simulink model "autopilota_v_15_last"  (R2020b)
settings: Solver=ode4  StartTime=0.0  StopTime=300  FixedStep=0.02  RelTol=1e-3
values from neighbouring files (symbols this model uses):
  attuatore_Amax = 20*(pi/180)    (= 0.349065850399)    [v2021_10_27_avvioSITL.m]    (also in v2021_10_27_calcoloAerodinamica.m)
  attuatore_Amin = -20*(pi/180)    (= -0.349065850399)    [v2021_10_27_avvioSITL.m]
  attuatore_Emax = 25*(pi/180)    (= 0.436332312999)    [v2021_10_27_avvioSITL.m]    (also in v2021_10_27_calcoloAerodinamica.m)
  attuatore_Emin = -25*(pi/180)    (= -0.436332312999)    [v2021_10_27_avvioSITL.m]
  attuatore_Rmax = 25*(pi/180)    (= 0.436332312999)    [v2021_10_27_avvioSITL.m]    (also in v2021_10_27_calcoloAerodinamica.m)
  attuatore_Rmin = -25*(pi/180)    (= -0.436332312999)    [v2021_10_27_avvioSITL.m]
  attuatore_Tmax = 0.99    [v2021_10_27_avvioSITL.m]
  attuatore_Tmin = 0    [v2021_10_27_avvioSITL.m]
  bias = [baccxINI,baccyINI,bacczINI,bpINI,bqINI,brINI]    [v2021_10_27_avvioSITL.m]
  final_h = 35    [v2021_10_27_avvioSITL.m]
  interventoA_05 = 20*0.8    (= 16)    [v2021_10_27_avvioSITL.m]
  interventoA_1 = 10    [v2021_10_27_avvioSITL.m]
  interventoE_05 = 25*0.8    (= 20)    [v2021_10_27_avvioSITL.m]
  interventoE_1 = 10    [v2021_10_27_avvioSITL.m]
  interventoT = 1*0.6    (= 0.6)    [v2021_10_27_avvioSITL.m]
  inv_A = 1    [v2021_10_27_avvioSITL.m]
  inv_comp_h = 1    [v2021_10_27_avvioSITL.m]
  inv_E = 1    [v2021_10_27_avvioSITL.m]
  inv_R = 1    [v2021_10_27_avvioSITL.m]
  inv_T = 1    [v2021_10_27_avvioSITL.m]
  K_AW_B_AP_quota = 1000    [v2021_10_27_avvioSITL.m]
  K_AW_B_becc = -250    [v2021_10_27_avvioSITL.m]
  K_AW_B_imb = 0    [v2021_10_27_avvioSITL.m]
  K_AW_B_roll = 500    [v2021_10_27_avvioSITL.m]
  K_imb_inv = -0.001306    [v2021_10_27_avvioSITL.m]
  Kd_AP_rotta = 0.995    [v2021_10_27_avvioSITL.m]
  Kd_h_app = 0.085    [v2021_10_27_avvioSITL.m]
  Kd_h_flare = 0.01    [v2021_10_27_avvioSITL.m]
  Ki_AP_quota_select = 0.01936    [v2021_10_27_avvioSITL.m]
  Ki_AP_rotta = 0.002    [v2021_10_27_avvioSITL.m]
  Ki_AP_vel = 0.025175    [v2021_10_27_avvioSITL.m]
  Ki_becch = -0.1963    [v2021_10_27_avvioSITL.m]
  Ki_h_app = 0.055    [v2021_10_27_avvioSITL.m]
  Ki_h_cruise = 0.008    [v2021_10_27_avvioSITL.m]
  Ki_h_flare = 0.07    [v2021_10_27_avvioSITL.m]
  Ki_roll = 0.004528    [v2021_10_27_avvioSITL.m]
  Kp_AP_quota_hold_h = 0.5503    [v2021_10_27_avvioSITL.m]
  Kp_AP_quota_hold_l = 0.5503    [v2021_10_27_avvioSITL.m]
  Kp_AP_quota_select = 0.02647    [v2021_10_27_avvioSITL.m]
  Kp_AP_rotta = 0.520    (= 0.52)    [v2021_10_27_avvioSITL.m]
  Kp_AP_vel = 0.132175    [v2021_10_27_avvioSITL.m]
  Kp_becch = -0.30    (= -0.3)    [v2021_10_27_avvioSITL.m]
  Kp_comp_h = 0.035    [v2021_10_27_avvioSITL.m]
  Kp_h_app_max = 0.086    [v2021_10_27_avvioSITL.m]
  Kp_h_app_min = 0.01    [v2021_10_27_avvioSITL.m]
  Kp_h_cruise = 0.04    [v2021_10_27_avvioSITL.m]
  Kp_h_flare = 0.1    [v2021_10_27_avvioSITL.m]
  Kp_imb = 0.0019415    [v2021_10_27_avvioSITL.m]
  Kp_p = 0.006913    [v2021_10_27_avvioSITL.m]
  Kp_q = -0.025    [v2021_10_27_avvioSITL.m]
  Kp_roll = 0.0718    [v2021_10_27_avvioSITL.m]
  Kp_Rotta_ATO = 4    [v2021_10_27_avvioSITL.m]
  Kp_Rotta_psi = -0.01    [v2021_10_27_avvioSITL.m]
  Q1B = [    2e-15;     2e-15 ... (first row only)    [COV_F1B.m]
  R1B = [     2e-14;             2e-14 ... (first row only)    [COV_F1B.m]
  safe_phi = 55    [v2021_10_27_avvioSITL.m]
  safe_V = 40    [v2021_10_27_avvioSITL.m]
  Sensor_Offsets = [0,0,0]    [v2021_10_27_avvioSITL.m]
  T_cal = 0.4    [v2021_10_27_avvioSITL.m]
  theta_rot = 10    [v2021_10_27_avvioSITL.m]
  time_alarm_SAFE = 300    [v2021_10_27_avvioSITL.m]
  tsamp = 0.02    [v2021_10_27_avvioSITL.m]
  update = [2,2,2]    [v2021_10_27_avvioSITL.m]
  V_max = 35    [v2021_10_27_avvioSITL.m]
  V_stall = 15    [v2021_10_27_avvioSITL.m]
  vd_ini = 0    [v2021_10_27_avvioSITL.m]
  vel_wp1_al = 25    [v2021_10_27_avvioSITL.m]
  vel_wp2_al = 20    [v2021_10_27_avvioSITL.m]
undefined symbols (not defined in the file or in its folder): DiscIntNeverNeededParam, Newton, Raphson, t_AP
libraries: simulink_extras x41, pid_lib x8, dspsigops x4, simulink x3, aerolibtransform2sys x2, aerolibtransform2 x2, cstblocks x1, aerosimlib x1
(part 2 of 11)

== system autopilota_v_15_last/MISURE DA SENSORI FILTRATE/initializer//Clk_generator 1 ==
  Misure : Inport
  calibrating : Inport  Port=2
  Gps_fix_3d : Inport  Port=3
  indice_di_mario : Inport  Port=4
  bias : Inport  Port=5
  Bus Selector2 : BusSelector  Commented=on  OutputSignals=Lat,Long,quota_baro,V_nord,V_est,phi,theta,psi,acc_x,acc_y,acc_z,p,q,r
  Clock GPS1 : Subsystem
  Clock Mti : Subsystem
  Constant : Constant  Value=vd_ini
  Constant1 : Constant
  Constant2 : Constant
  Display : Display
      settings: Decimation=4
  In1 : InportShadow  Port=2
  MATLAB Function2 : MATLAB Function  TreatAsAtomicUnit=on
  Mux2 : Mux  Commented=on  Inputs=14
  Sample and Hold : dspsigops/Sample and Hold  trig=Rising edge  initCond=0  latchinput=off
  Scope2 : Scope  NumInputPorts=3
  Scope3 : Scope  NumInputPorts=2
  Step : Step  Time=T_cal  SampleTime=0.02
  Switch : Switch  Criteria=u2 > Threshold
  Terminator : Terminator
  Cond_ini : Outport  VectorParamsAs1DForOutWhenUnconnected=off
  Enable : Outport  Port=2  VectorParamsAs1DForOutWhenUnconnected=off
  CLock_gps_pos : Outport  Port=3  VectorParamsAs1DForOutWhenUnconnected=off
  "Clock_gps_vel " : Outport  Port=4  VectorParamsAs1DForOutWhenUnconnected=off
  CLock_mti : Outport  Port=5  VectorParamsAs1DForOutWhenUnconnected=off
  wires:
  Gps_fix_3d/1 -> MATLAB Function2/5(fix)
  Clock GPS1/1(clk_pos) -> MATLAB Function2/3(clk_gps), CLock_gps_pos/1, Scope2/2
  Clock Mti/1(Out1) -> Scope2/3, CLock_mti/1, MATLAB Function2/2(clk_ahrs)
  Constant/1 -> MATLAB Function2/6(vd_ini)
  bias/1 -> MATLAB Function2/7(bias)
  indice_di_mario/1 -> Clock GPS1/1(In1)
  Bus Selector2/1 -> Mux2/1  "<Lat>"
  Bus Selector2/2 -> Mux2/2  "<Long>"
  Bus Selector2/3 -> Mux2/3  "<quota_baro>"
  Bus Selector2/4 -> Mux2/4  "<V_nord>"
  Bus Selector2/5 -> Mux2/5  "<V_est>"
  Bus Selector2/6 -> Mux2/6  "<phi>"
  Bus Selector2/7 -> Mux2/7  "<theta>"
  Bus Selector2/8 -> Mux2/8  "<psi>"
  Bus Selector2/9 -> Mux2/9  "<acc_x>"
  Bus Selector2/10 -> Mux2/10  "<acc_y>"
  Bus Selector2/11 -> Mux2/11  "<acc_z>"
  Bus Selector2/12 -> Mux2/12  "<p>"
  Bus Selector2/13 -> Mux2/13  "<q>"
  Bus Selector2/14 -> Mux2/14  "<r>"
  calibrating/1 -> MATLAB Function2/4(Calibrating)
  Step/1 -> Scope3/1
  In1/1 -> Switch/3
  Constant1/1 -> Switch/1
  Switch/1 -> Scope3/2, Enable/1, Sample and Hold/Trigger
  Misure/1 -> Clock Mti/1(In2), Clock GPS1/2(In2), MATLAB Function2/1(misure)
  Clock GPS1/2(clk_vel) -> Scope2/1, "Clock_gps_vel "/1
  MATLAB Function2/1(y) -> Sample and Hold/1
  Sample and Hold/1 -> Display/1, Cond_ini/1
  MATLAB Function2/2(en) -> Terminator/1
  Constant2/1 -> Switch/2

== system autopilota_v_15_last/MISURE DA SENSORI FILTRATE SENZA KALMAN/AOA1 ==
  theta : Inport
  Tas : Inport  Port=2
  RC : Inport  Port=3
  Divide : Product  Inputs=*/
  Sum1 : Sum  Inputs=+-|
  Trigonometric Function : Trigonometry  Operator=asin
  AOA : Outport  VectorParamsAs1DForOutWhenUnconnected=off
  wires:
  theta/1 -> Sum1/1
  Divide/1 -> Trigonometric Function/1
  Sum1/1 -> AOA/1
  Tas/1 -> Divide/2
  Trigonometric Function/1 -> Sum1/2
  RC/1 -> Divide/1

== system autopilota_v_15_last/MISURE DA SENSORI FILTRATE SENZA KALMAN/Subsystem ==
  0-360 : Inport
  Constant : Constant  Value=360
  Sum : Sum  Inputs=|+-
  Switch : Switch  Criteria=u2 > Threshold  Threshold=180
  "+-180 " : Outport  VectorParamsAs1DForOutWhenUnconnected=off
  wires:
  Switch/1 -> "+-180 "/1
  Constant/1 -> Sum/2
  Sum/1 -> Switch/1
  0-360/1 -> Sum/1, Switch/3, Switch/2

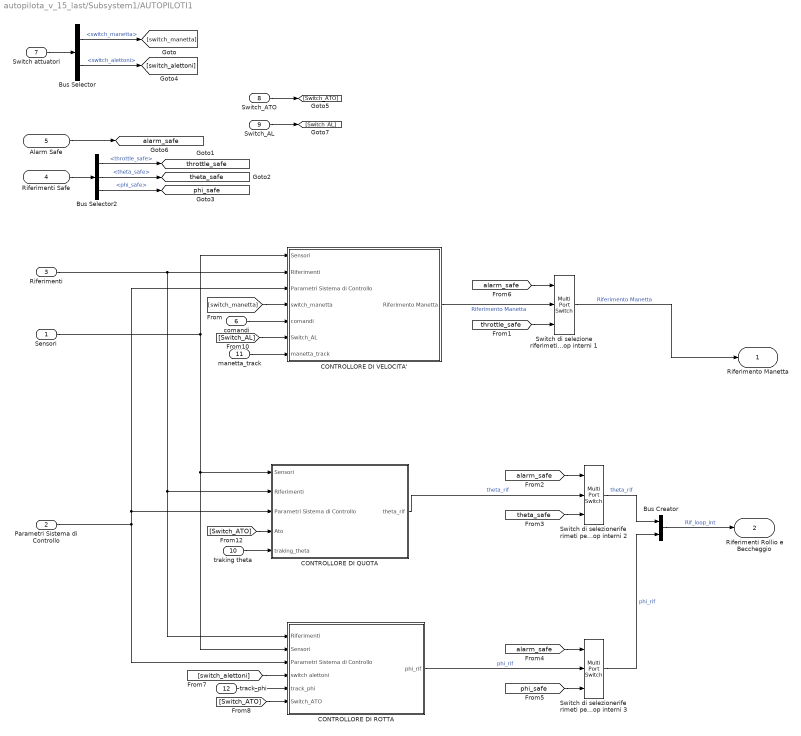
== system autopilota_v_15_last/Subsystem1/AUTOPILOTI1 ==
  Sensori : Inport
  Parametri Sistema di Controllo : Inport  Port=2
  Riferimenti : Inport  Port=3
  Riferimenti Safe : Inport  Port=4
  Alarm Safe : Inport  Port=5
  comandi : Inport  Port=6
  Switch attuatori : Inport  Port=7
  Switch_ATO : Inport  Port=8
  Switch_AL : Inport  Port=9
  traking theta : Inport  Port=10
  manetta_track : Inport  Port=11
  track_phi : Inport  Port=12
  Bus Creator : BusCreator  Inputs=2
  Bus Selector : BusSelector  OutputSignals=switch_manetta,switch_alettoni
  Bus Selector2 : BusSelector  OutputSignals=throttle_safe,theta_safe,phi_safe
  CONTROLLORE DI QUOTA : Subsystem
  CONTROLLORE DI ROTTA : Subsystem
  CONTROLLORE DI VELOCITA' : Subsystem
  Switch di selezione riferimeti per i loop interni 1 : MultiPortSwitch  DataPortOrder=Zero-based contiguous  Inputs=2  zeroidx=on
  Switch di selezioneriferimeti per i loop interni 2 : MultiPortSwitch  DataPortOrder=Zero-based contiguous  Inputs=2  zeroidx=on
  Switch di selezioneriferimeti per i loop interni 3 : MultiPortSwitch  DataPortOrder=Zero-based contiguous  Inputs=2  zeroidx=on
  Riferimento Manetta : Outport  VectorParamsAs1DForOutWhenUnconnected=off
  Riferimenti Rollio e Beccheggio : Outport  Port=2  VectorParamsAs1DForOutWhenUnconnected=off
  tag scope: alarm_safe=global, phi_safe=global, theta_safe=global, throttle_safe=global
  wires:
  Bus Creator/1 -> Riferimenti Rollio e Beccheggio/1  "Rif_loop_int"
  CONTROLLORE DI VELOCITA'/1(Riferimento Manetta) -> Switch di selezione riferimeti per i loop interni 1/2  "Riferimento Manetta"
  Switch di selezione riferimeti per i loop interni 1/1 -> Riferimento Manetta/1  "Riferimento Manetta"
  Switch di selezioneriferimeti per i loop interni 2/1 -> Bus Creator/1  "theta_rif"
  Switch di selezioneriferimeti per i loop interni 3/1 -> Bus Creator/2  "phi_rif"
  [alarm_safe] -> Switch di selezioneriferimeti per i loop interni 2/1
  [alarm_safe] -> Switch di selezioneriferimeti per i loop interni 3/1
  Sensori/1 -> CONTROLLORE DI VELOCITA'/1(Sensori), CONTROLLORE DI ROTTA/2(Sensori), CONTROLLORE DI QUOTA/1(Sensori)
  Riferimenti/1 -> CONTROLLORE DI ROTTA/1(Riferimenti), CONTROLLORE DI QUOTA/2(Riferimenti), CONTROLLORE DI VELOCITA'/2(Riferimenti)
  Parametri Sistema di Controllo/1 -> CONTROLLORE DI VELOCITA'/3(Parametri Sistema di Controllo), CONTROLLORE DI QUOTA/3(Parametri Sistema di Controllo), CONTROLLORE DI ROTTA/3(Parametri Sistema di Controllo)
  Riferimenti Safe/1 -> Bus Selector2/1
  Alarm Safe/1 -> [alarm_safe]
  Bus Selector2/1 -> [throttle_safe]  "<throttle_safe>"
  Bus Selector2/2 -> [theta_safe]  "<theta_safe>"
  Bus Selector2/3 -> [phi_safe]  "<phi_safe>"
  [alarm_safe] -> Switch di selezione riferimeti per i loop interni 1/1
  [throttle_safe] -> Switch di selezione riferimeti per i loop interni 1/3
  [theta_safe] -> Switch di selezioneriferimeti per i loop interni 2/3
  [phi_safe] -> Switch di selezioneriferimeti per i loop interni 3/3
  Switch attuatori/1 -> Bus Selector/1
  Bus Selector/1 -> [switch_manetta]  "<switch_manetta>"
  Bus Selector/2 -> [switch_alettoni]  "<switch_alettoni>"
  comandi/1 -> CONTROLLORE DI VELOCITA'/5(comandi)
  [switch_manetta] -> CONTROLLORE DI VELOCITA'/4(switch_manetta)
  [switch_alettoni] -> CONTROLLORE DI ROTTA/4("switch alettoni ")
  CONTROLLORE DI ROTTA/1(phi_rif) -> Switch di selezioneriferimeti per i loop interni 3/2  "phi_rif"
  Switch_ATO/1 -> [Switch_ATO]
  Switch_AL/1 -> [Switch_AL]
  [Switch_AL] -> CONTROLLORE DI VELOCITA'/6(Switch_AL)
  CONTROLLORE DI QUOTA/1(theta_rif) -> Switch di selezioneriferimeti per i loop interni 2/2  "theta_rif"
  [Switch_ATO] -> CONTROLLORE DI QUOTA/4(Ato)
  traking theta/1 -> CONTROLLORE DI QUOTA/5(traking_theta)
  manetta_track/1 -> CONTROLLORE DI VELOCITA'/7(manetta_track)
  track_phi/1 -> CONTROLLORE DI ROTTA/5(track_phi)
  [Switch_ATO] -> CONTROLLORE DI ROTTA/6(Switch_ATO)

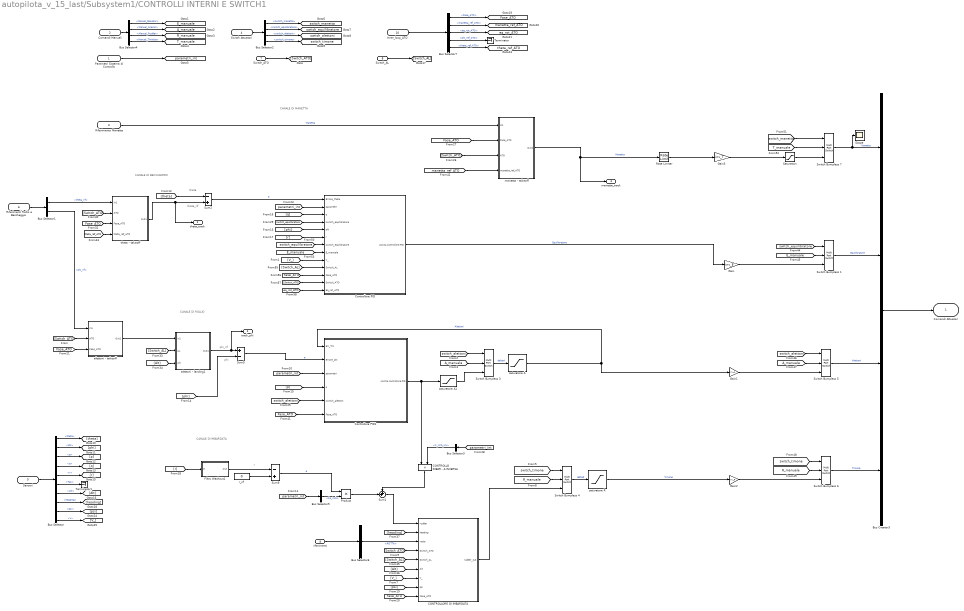
== system autopilota_v_15_last/Subsystem1/CONTROLLI INTERNI E SWITCH1 ==
  note: CANALE DI
      |  MANETTA
  note: theta
  note: theta_rif
  note: CANALE DI
      |  BECCHEGGIO
  note: CANALE
      | DI ROLLIO
  note: CANALE
      | DI IMBARDATA
  note: phi
  note: phi_rif
  note: r
  Parametri Sistema di Controllo : Inport
  Comandi Manuali : Inport  Port=2
  Riferimento Manetta : Inport  Port=3
  Switch Attuatori : Inport  Port=4
  Sensori : Inport  Port=5
  Riferimenti Rollio e Beccheggio : Inport  Port=6
  Switch_ATO : Inport  Port=7
  Switch_AL : Inport  Port=8
  riferimenti : Inport  Port=9
  Inner_loop_ATO : Inport  Port=10
  "  CONTROLLO IMBARDATA INVERSA" : Product  RndMeth=Zero
  Bus Creator3 : BusCreator  Inputs=4
  Bus Selector : BusSelector  OutputSignals=theta,phi,p,q,r,Tas,Alt,heading,psi,v
  Bus Selector1 : BusSelector  OutputSignals=theta_rif,phi_rif
  Bus Selector2 : BusSelector  OutputSignals=switch_manetta,switch_equilibratore,switch_alettoni,switch_timone
  Bus Selector3 : BusSelector  OutputSignals=K_imb_inv
  Bus Selector4 : BusSelector  OutputSignals=Manual_Elevator,Manual_Aileron,Manual_Rudder,Manual_Throttle
  Bus Selector5 : BusSelector  OutputSignals=Kp_imb
  Bus Selector6 : BusSelector  OutputSignals=ROTTA
  Bus Selector7 : BusSelector  OutputSignals=Fase_ATO,manetta_ref_ATO,eq_rot_ATO,phi_ref_ATO,theta_ref_ATO
  CONTROLLORE DI IMBARDATA : Subsystem
  Controllore PID : Subsystem
  Controllore PID1 : Subsystem
  Filtro Washout1 : Subsystem
  Gain : Gain  Gain=inv_E
  Gain1 : Gain  Gain=inv_A
  Gain2 : Gain  Gain=inv_R
  Gain3 : Gain  Gain=inv_T
  Product : Product  RndMeth=Zero
  Rate Limiter : RateLimiter  RisingSlewLimit=0.3  FallingSlewLimit=-0.3  SampleTimeMode=inherited
  Saturation : Saturate  UpperLimit=attuatore_Tmax  LowerLimit=attuatore_Tmin
  Scope : Scope
  Sum1 : Sum  Inputs=++|
  Sum2 : Sum  Inputs=-+
  Sum5 : Sum  Inputs=+-
  Sum9 : Sum  Inputs=-+
  Switch Bumpless {1,3..7} (6 alike) : MultiPortSwitch  DataPortOrder=Zero-based contiguous  Inputs=2  zeroidx=on
  Terminator : Terminator
  Terminator1 : Terminator
  alettoni - landing1 : Subsystem
  alettoni - takeoff : Subsystem
  manetta - takeoff : Subsystem
  r_rif : Constant  Value=0  SampleTime=t_AP
  saturatore A : Saturate  UpperLimit=attuatore_Amax  LowerLimit=attuatore_Amin
  saturatore A1 : Saturate  UpperLimit=attuatore_Amax  LowerLimit=attuatore_Amin
  saturatore R : Saturate  UpperLimit=attuatore_Rmax  LowerLimit=attuatore_Rmin
  theta - takeoff : Subsystem
  Comandi Attuatori : Outport  VectorParamsAs1DForOutWhenUnconnected=off
  theta_track : Outport  Port=2  VectorParamsAs1DForOutWhenUnconnected=off
  manetta_track : Outport  Port=3  VectorParamsAs1DForOutWhenUnconnected=off
  track_phi : Outport  Port=4  VectorParamsAs1DForOutWhenUnconnected=off
  tag scope: A_manuale=global, E_manuale=global, Fase_ATO=global, R_manuale=global, T_manuale=global, eq_rot_ATO=global, manetta_ref_ATO=global, parametri_int=global, switch_alettoni=global, switch_equilibratore=global, switch_manetta=global, switch_timone=global, theta_ref_ATO=global
  wires:
  Comandi Manuali/1 -> Bus Selector4/1
  Bus Selector4/1 -> [E_manuale]  "<Manual_Elevator>"
  Bus Selector4/2 -> [A_manuale]  "<Manual_Aileron>"
  Bus Selector4/3 -> [R_manuale]  "<Manual_Rudder>"
  Bus Selector4/4 -> [T_manuale]  "<Manual_Throttle>"
  Parametri Sistema di Controllo/1 -> [parametri_int]
  Switch Attuatori/1 -> Bus Selector2/1
  Bus Selector2/1 -> [switch_manetta]  "<switch_manetta>"
  Bus Selector2/2 -> [switch_equilibratore]  "<switch_equilibratore>"
  Bus Selector2/3 -> [switch_alettoni]  "<switch_alettoni>"
  Bus Selector2/4 -> [switch_timone]  "<switch_timone>"
  Sensori/1 -> Bus Selector/1
  Riferimenti Rollio e Beccheggio/1 -> Bus Selector1/1
  Bus Selector1/2 -> alettoni - takeoff/1(In1)  "<phi_rif>"
  Switch Bumpless 3/1 -> saturatore A/1  "deltaA"
  saturatore A/1 -> Gain1/1, Controllore PID1/1(Err_Trk)  "Alettoni"
  [switch_alettoni] -> Switch Bumpless 3/1
  [A_manuale] -> Switch Bumpless 3/2
  [switch_timone] -> Switch Bumpless 4/1
  [R_manuale] -> Switch Bumpless 4/2
  r_rif/1 -> Sum9/2
  Filtro Washout1/1(Out) -> Sum9/1
  Bus Creator3/1 -> Comandi Attuatori/1
  Bus Selector3/1 -> "  CONTROLLO IMBARDATA INVERSA"/2  "<K_imb_inv>"
  [parametri_int] -> Bus Selector3/1
  Sum2/1 -> Controllore PID/1(Errore_theta)  "e"
  [switch_equilibratore] -> Controllore PID/4("switch_equilibratore ")
  saturatore A1/1 -> Switch Bumpless 3/3
  [parametri_int] -> Controllore PID/2(parametri)
  [parametri_int] -> Controllore PID1/3(parametri)
  Sum5/1 -> Controllore PID1/2(Errore_phi)  "e"
  Controllore PID1/1(Uscita controllore PID) -> "  CONTROLLO IMBARDATA INVERSA"/1, saturatore A1/1
  saturatore R/1 -> Gain2/1  "Timone"
  Switch Bumpless 4/1 -> saturatore R/1  "deltaR"
  Sum9/1 -> Product/1  "e"
  [parametri_int] -> Bus Selector5/1
  Bus Selector5/1 -> Product/2  "<Kp_imb>"
  Product/1 -> Sum1/2
  Sum1/1 -> CONTROLLORE DI IMBARDATA/1(rudder)
  "  CONTROLLO IMBARDATA INVERSA"/1 -> Sum1/1
  Switch_ATO/1 -> [Switch_ATO]
  Bus Selector/6 -> Terminator1/1  "<Tas>"
  Bus Selector/7 -> [Alt]  "<Alt>"
  alettoni - takeoff/1(Out1) -> alettoni - landing1/1(In1)
  [V_] -> CONTROLLORE DI IMBARDATA/7(V_)
  [Switch_ATO] -> CONTROLLORE DI IMBARDATA/4(Switch_ATO)
  CONTROLLORE DI IMBARDATA/1(rudder_out) -> Switch Bumpless 4/3
  Switch_AL/1 -> [Switch_AL]
  Controllore PID/1(Uscita controllore PID) -> Gain/1  "Equilibratore"
  alettoni - landing1/1(Out1) -> track_phi/1, Sum5/1
  [Switch_AL] -> alettoni - landing1/2(AL)
  [Alt] -> alettoni - landing1/3(Alt)
  [Switch_AL] -> CONTROLLORE DI IMBARDATA/5(Switch_AL)
  [Alt] -> CONTROLLORE DI IMBARDATA/6(Alt)
  riferimenti/1 -> Bus Selector6/1
  Bus Selector6/1 -> CONTROLLORE DI IMBARDATA/3(rotta)  "<ROTTA>"
  [heading] -> CONTROLLORE DI IMBARDATA/2(heading)
  Inner_loop_ATO/1 -> Bus Selector7/1
  Bus Selector7/1 -> [Fase_ATO]  "<Fase_ATO>"
  Bus Selector7/2 -> [manetta_ref_ATO]  "<manetta_ref_ATO>"
  Bus Selector7/3 -> [eq_rot_ATO]  "<eq_rot_ATO>"
  Bus Selector7/4 -> Terminator/1  "<phi_ref_ATO>"
  Bus Selector7/5 -> [theta_ref_ATO]  "<theta_ref_ATO>"
  manetta - takeoff/1(Out1) -> Rate Limiter/1, manetta_track/1  "Manetta"
  Riferimento Manetta/1 -> manetta - takeoff/1(In1)  "Manetta"
  [switch_alettoni] -> Controllore PID1/5("switch_alettoni ")
  [theta] -> Sum2/1
  Bus Selector/1 -> [theta]  "<theta>"
  [phi] -> Controllore PID/5("phi ")
  [phi] -> Sum5/2
  Bus Selector/2 -> [phi]  "<phi>"
  [p] -> Controllore PID1/4("p ")
  Bus Selector/3 -> [p]  "<p>"
  [q] -> Controllore PID/3("q ")
  Bus Selector/4 -> [q]  "<q>"
  [r] -> Controllore PID/6(r)
  [r] -> Filtro Washout1/1(In)
  Bus Selector/5 -> [r]  "<r>"
  Bus Selector/9 -> [psi]  "<psi>"
  [psi] -> CONTROLLORE DI IMBARDATA/8(psi)
  [Fase_ATO] -> CONTROLLORE DI IMBARDATA/9(Fase_ATO)
  [Switch_ATO] -> alettoni - takeoff/2(ATO)
  [Fase_ATO] -> alettoni - takeoff/3(Fase_ATO)
  [Switch_ATO] -> manetta - takeoff/3(ATO)
  [Fase_ATO] -> manetta - takeoff/2(Fase_ATO)
  [manetta_ref_ATO] -> manetta - takeoff/4(manetta_ref_ATO)
  Bus Selector1/1 -> theta - takeoff/1(In1)  "<theta_rif>"
  [Switch_ATO] -> theta - takeoff/2(ATO)
  [Fase_ATO] -> theta - takeoff/3(Fase_ATO)
  [Fase_ATO] -> Controllore PID1/6(Fase_ATO)
  Bus Selector/8 -> [heading]  "<heading>"
  [theta_ref_ATO] -> theta - takeoff/4(theta_ref_ATO)
  Bus Selector/10 -> [V_]  "<v>"
  theta - takeoff/1(Out1) -> theta_track/1, Sum2/2
  Switch Bumpless 1/1 -> Bus Creator3/2  "Equilibratore"
  [E_manuale] -> Switch Bumpless 1/2
  [switch_equilibratore] -> Switch Bumpless 1/1
  Gain/1 -> Switch Bumpless 1/3
  [switch_alettoni] -> Switch Bumpless 5/1
  [A_manuale] -> Switch Bumpless 5/2
  Switch Bumpless 5/1 -> Bus Creator3/3  "Alettoni"
  Gain1/1 -> Switch Bumpless 5/3
  [switch_timone] -> Switch Bumpless 6/1
  [R_manuale] -> Switch Bumpless 6/2
  Switch Bumpless 6/1 -> Bus Creator3/4  "Timone"
  Gain2/1 -> Switch Bumpless 6/3
  [switch_manetta] -> Switch Bumpless 7/1
  [T_manuale] -> Switch Bumpless 7/2
  Switch Bumpless 7/1 -> Scope/1, Bus Creator3/1  "Manetta"
  Gain3/1 -> Saturation/1
  [switch_equilibratore] -> Controllore PID/7(switch_equilibratore)
  [E_manuale] -> Controllore PID/8(E_manuale)
  [Switch_AL] -> Controllore PID/10(Switch_AL)
  [V_] -> Controllore PID/9(V_)
  [Fase_ATO] -> Controllore PID/11(Fase_ATO)
  [Switch_ATO] -> Controllore PID/12(Switch_ATO)
  [eq_rot_ATO] -> Controllore PID/13(Eq_rot_ATO)
  Rate Limiter/1 -> Gain3/1
  Saturation/1 -> Switch Bumpless 7/3

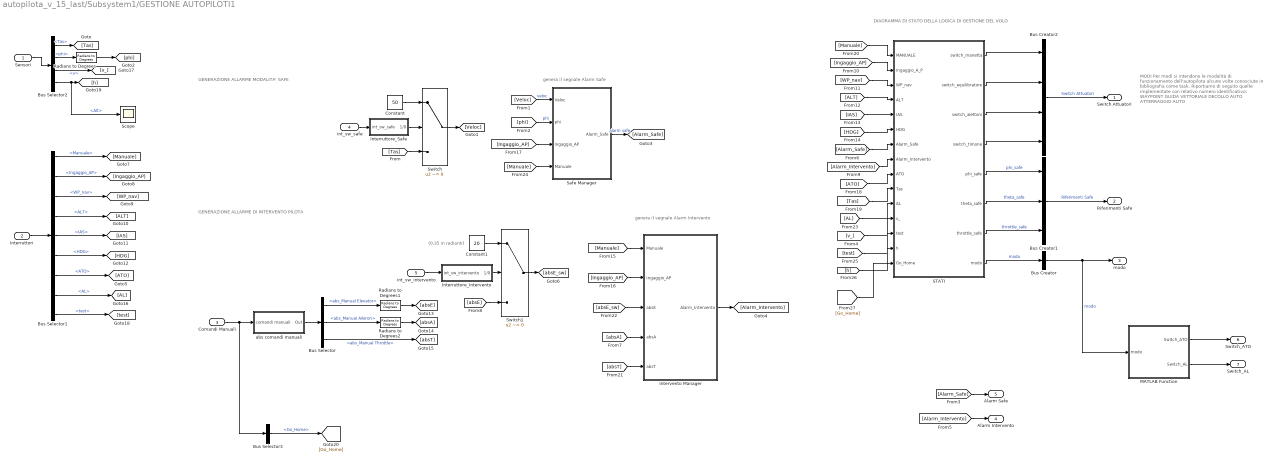
== system autopilota_v_15_last/Subsystem1/GESTIONE AUTOPILOTI1 ==
  note: (0.35 in radianti)
  note: GENERAZIONE ALLARME DI INTERVENTO PILOTA
  note: genera il segnale Alarm Safe
  note: genera il segnale Alarm Intervento
  note: GENERAZIONE ALLARME MODALITA' SAFE
  note: DIAGRAMMA DI STATO
      | DELLA LOGICA DI GESTIONE DEL VOLO
  note: MODI
      | Per modi si intendono le modalità di funzionamento dell'autopilota alcune volte conosciute in bibliografia come task. Riportiamo di seguito quelle implementate con relativo numero identificativo:
      |
      | WAYPOINT
      | GUIDA VETTORIALE
      | DECOLLO AUTO
      | ATTERRAGGIO AUTO
  Sensori : Inport
  "Interruttori " : Inport  Port=2
  Comandi Manuali : Inport  Port=3
  int_sw_safe : Inport  Port=4
  int_sw_intervento : Inport  Port=5
  " STATI" : Stateflow chart  TreatAsAtomicUnit=on
  Bus Creator : BusCreator  Inputs=1
  Bus Creator1 : BusCreator  Inputs=3
  Bus Creator2 : BusCreator  Inputs=4
  Bus Selector : BusSelector  OutputSignals=abs_Manual Elevator,abs_Manual Aileron,abs_Manual Throttle
  Bus Selector1 : BusSelector  OutputSignals=Manuale,Ingaggio_AP,WP_nav,ALT,IAS,HDG,ATO,AL,test
  Bus Selector2 : BusSelector  OutputSignals=Tas,phi,v,Alt
  Bus Selector3 : BusSelector  OutputSignals=Go_Home
  Constant : Constant  Value=50
  Constant1 : Constant  Value=20
  Interruttore_Intervento : Subsystem
  Interruttore_Safe : Subsystem
  Intervento Manager : Subsystem
  MATLAB Function : MATLAB Function  TreatAsAtomicUnit=on
  Radians to Degrees : simulink_extras/Transformations/Radians to Degrees
  Radians to Degrees1 : simulink_extras/Transformations/Radians to Degrees
  Radians to Degrees2 : simulink_extras/Transformations/Radians to Degrees
  Safe Manager : Subsystem
  Scope : Scope
  Switch : Switch  Criteria=u2 ~= 0
  Switch1 : Switch  Criteria=u2 ~= 0
  abs comandi manuali : Subsystem
  Switch Attuatori : Outport  VectorParamsAs1DForOutWhenUnconnected=off
  Riferimenti Safe : Outport  Port=2  VectorParamsAs1DForOutWhenUnconnected=off
  modo : Outport  Port=3  VectorParamsAs1DForOutWhenUnconnected=off
  Alarm Intervento : Outport  Port=4  VectorParamsAs1DForOutWhenUnconnected=off
  Alarm Safe : Outport  Port=5  VectorParamsAs1DForOutWhenUnconnected=off
  Switch_ATO : Outport  Port=6  VectorParamsAs1DForOutWhenUnconnected=off
  Switch_AL : Outport  Port=7  VectorParamsAs1DForOutWhenUnconnected=off
  wires:
  "Interruttori "/1 -> Bus Selector1/1
  Bus Selector1/1 -> [Manuale]  "<Manuale>"
  abs comandi manuali/1(Out) -> Bus Selector/1
  Bus Selector/1 -> Radians to Degrees1/1  "<abs_Manual Elevator>"
  Bus Selector/3 -> [absT]  "<abs_Manual Throttle>"
  Comandi Manuali/1 -> Bus Selector3/1, abs comandi manuali/1(comandi manuali)
  Sensori/1 -> Bus Selector2/1
  Bus Selector1/4 -> [ALT]  "<ALT>"
  Bus Selector1/5 -> [IAS]  "<IAS>"
  Bus Selector1/6 -> [HDG]  "<HDG>"
  Bus Selector2/2 -> Radians to Degrees/1  "<phi>"
  Radians to Degrees/1 -> [phi]
  Bus Selector/2 -> Radians to Degrees2/1  "<abs_Manual Aileron>"
  Bus Selector1/3 -> [WP_nav]  "<WP_nav>"
  Bus Selector2/1 -> [Tas]  "<Tas>"
  Switch/1 -> [Veloc]
  Constant/1 -> Switch/1
  [Tas] -> Switch/3
  [Veloc] -> Safe Manager/1(Veloc)  "veloc"
  Bus Selector1/2 -> [Ingaggio_AP]  "<Ingaggio_AP>"
  [phi] -> Safe Manager/2(phi)  "phi"
  Interruttore_Safe/1(1/0) -> Switch/2
  [Alarm_Safe] -> Alarm Safe/1
  Intervento Manager/1(Alarm_Intervento) -> [Alarm_Intervento]
  [Alarm_Intervento] -> Alarm Intervento/1
  Constant1/1 -> Switch1/1
  [absE] -> Switch1/3
  int_sw_intervento/1 -> Interruttore_Intervento/1(int_sw_intervento)
  Interruttore_Intervento/1(1/0) -> Switch1/2
  [Manuale] -> Intervento Manager/1(Manuale)
  [Ingaggio_AP] -> Intervento Manager/2(Ingaggio_AP)
  [Ingaggio_AP] -> Safe Manager/3(ingaggio_AP)
  [absA] -> Intervento Manager/4(absA)
  int_sw_safe/1 -> Interruttore_Safe/1(int_sw_safe)
  Switch1/1 -> [absE_sw]
  [absE_sw] -> Intervento Manager/3(absE)
  Radians to Degrees1/1 -> [absE]
  Radians to Degrees2/1 -> [absA]
  [absT] -> Intervento Manager/5(absT)
  Bus Selector1/7 -> [ATO]  "<ATO>"
  " STATI"/5(phi_safe) -> Bus Creator1/1  "phi_safe"
  " STATI"/6(theta_safe) -> Bus Creator1/2  "theta_safe"
  " STATI"/7(throttle_safe) -> Bus Creator1/3  "throttle_safe"
  Bus Creator1/1 -> Riferimenti Safe/1  "Riferimenti Safe"
  " STATI"/1(switch_manetta) -> Bus Creator2/1
  " STATI"/2(switch_equilibratore) -> Bus Creator2/2
  " STATI"/3(switch_alettoni) -> Bus Creator2/3
  " STATI"/4(switch_timone) -> Bus Creator2/4
  Bus Creator2/1 -> Switch Attuatori/1  "Switch Attuatori"
  " STATI"/8(modo) -> Bus Creator/1  "modo"
  Bus Creator/1 -> MATLAB Function/1(modo), modo/1  "modo"
  [Alarm_Safe] -> " STATI"/7(Alarm_Safe)
  [Alarm_Intervento] -> " STATI"/8(Alarm_Intervento)
  [Manuale] -> " STATI"/1(MANUALE)
  [Ingaggio_AP] -> " STATI"/2(Ingaggio_A_P)
  [WP_nav] -> " STATI"/3(WP_nav)
  [ALT] -> " STATI"/4(ALT)
  [IAS] -> " STATI"/5(IAS)
  [HDG] -> " STATI"/6(HDG)
  [ATO] -> " STATI"/9(ATO)
  [Tas] -> " STATI"/10(Tas)
  Bus Selector1/8 -> [AL]  "<AL>"
  [AL] -> " STATI"/11(AL)
  Bus Selector2/3 -> [v_]  "<v>"
  [v_] -> " STATI"/12(v_)
  [Manuale] -> Safe Manager/4(Manuale)
  Bus Selector1/9 -> [test]  "<test>"
  [test] -> " STATI"/13(test)
  MATLAB Function/1(Switch_ATO) -> Switch_ATO/1
  MATLAB Function/2(Switch_AL) -> Switch_AL/1
  Bus Selector2/4 -> Scope/1, [h]  "<Alt>"
  [h] -> " STATI"/14(h)
  Bus Selector3/1 -> [Go_Home]  "<Go_Home>"
  [Go_Home] -> " STATI"/15(Go_Home)
  Safe Manager/1(Alarm_Safe) -> [Alarm_Safe]  "alarm safe"

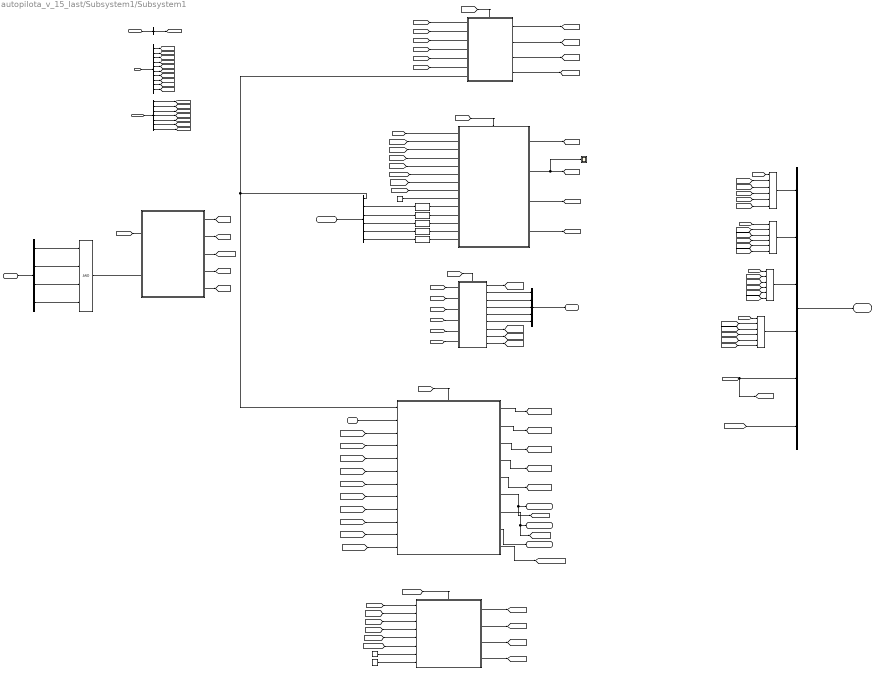
== system autopilota_v_15_last/Subsystem1/Subsystem1 ==
  note: MODO 1 : WAYPOINTS
  note: MODO 2 : VETTORIALE
  note: MODO 3 : DECOLLO AUTO
  note: MODO 4 : ATTERRAGGIO AUTO
  note: MODO 5 : GO HOME
  sensori : Inport
  Interruttori : Inport  Port=2
  waypoints e riferimenti vettoriali : Inport  Port=3
  modo : Inport  Port=4
  Cal_Home : Inport  Port=5
  Switch_attuatori : Inport  Port=6
  AND : Logic  Inputs=4  IconShape=distinctive  AllPortsSameDT=off  OutDataTypeStr=boolean
  Bus Creator : BusCreator  Inputs=5
  Bus Creator2 : BusCreator  Inputs=6
  Bus Selector : BusSelector  OutputSignals=Lat,Long,Alt,psi,heading,Tas,v,theta,RC,quota_lidar
  Bus Selector1 : BusSelector  OutputSignals=GC_info,IAS,ALT,HDG,RC,Ingaggio_AP
  Bus Selector2 : BusSelector  OutputSignals=WP_db_param,WP_db_info,ROTTA,VELOCITA,QUOTA,RC,WP_AL
  Bus Selector3 : BusSelector  OutputSignals=modo
  Bus Selector4 : BusSelector  OutputSignals=switch_manetta,switch_equilibratore,switch_alettoni,switch_timone
  Chart : Stateflow chart  TreatAsAtomicUnit=on
  Constant : Constant  Value=70
  Constant1 : Constant  Value=20
  DECOLLO AUTOMATICO : Subsystem
  Data Type Conversion{,1..4} (5 alike) : DataTypeConversion  OutDataTypeStr=uint8
  RC_default : Constant  Value=2  SampleTime=t_AP
  Scope : Scope
  Subsystem : Subsystem
  Subsystem1 : Subsystem
  Subsystem2 : Subsystem
  Subsystem3 : Subsystem
  Switch di selezione Task - Waypoint navigation{,1..3} (4 alike) : MultiPortSwitch  Inputs=5
  Riferimenti : Outport  VectorParamsAs1DForOutWhenUnconnected=off
  Inner_loop_ATO : Outport  Port=2  VectorParamsAs1DForOutWhenUnconnected=off
  H_LAT : Outport  Port=3  VectorParamsAs1DForOutWhenUnconnected=off
  H_LONG : Outport  Port=4  VectorParamsAs1DForOutWhenUnconnected=off
  H_ALT : Outport  Port=5  VectorParamsAs1DForOutWhenUnconnected=off
  tag scope: modo=global, selector_AL=global
  wires:
  waypoints e riferimenti vettoriali/1 -> Bus Selector2/1
  Bus Selector2/3 -> [ROTTA]  "<ROTTA>"
  Bus Selector2/4 -> [VELOCITA]  "<VELOCITA>"
  Bus Selector2/5 -> [QUOTA]  "<QUOTA>"
  Bus Selector2/6 -> [RC]  "<RC>"
  modo/1 -> Bus Selector3/1
  Bus Selector2/1 -> [WP_db_param]  "<WP_db_param>"
  Bus Selector2/2 -> [WP_db_info]  "<WP_db_info>"
  sensori/1 -> Bus Selector/1
  Bus Selector/1 -> [Lat]  "<Lat>"
  Bus Selector/2 -> [Long]  "<Long>"
  Bus Selector/3 -> [h]  "<Alt>"
  Bus Selector/4 -> [psi]  "<psi>"
  Bus Selector3/1 -> [modo]  "<modo>"
  Bus Selector/6 -> [Tas]  "<Tas>"
  [Tas] -> DECOLLO AUTOMATICO/1(Tas)
  DECOLLO AUTOMATICO/1(rotta_ATO) -> [rotta_ATO]
  DECOLLO AUTOMATICO/7(h_ref_ATO) -> [h_ATO]
  DECOLLO AUTOMATICO/9(RC_ref_ATO) -> [RC_ATO]
  DECOLLO AUTOMATICO/8(Tas_ref_ATO) -> [V_ATO]
  Interruttori/1 -> Bus Selector1/1
  Bus Selector2/7 -> [WP_AL]  "<WP_AL>"
  Bus Selector/7 -> [V_]  "<v>"
  Switch di selezione Task - Waypoint navigation3/1 -> Bus Creator2/4  "ROTTA"
  Bus Creator2/1 -> Riferimenti/1
  Switch di selezione Task - Waypoint navigation/1 -> Bus Creator2/1  "RC"
  Switch di selezione Task - Waypoint navigation1/1 -> Bus Creator2/2  "VELOCITA"
  [modo] -> Switch di selezione Task - Waypoint navigation/1
  [modo] -> Switch di selezione Task - Waypoint navigation1/1
  [modo] -> Switch di selezione Task - Waypoint navigation2/1
  [modo] -> Switch di selezione Task - Waypoint navigation3/1
  [RC_vett] -> Switch di selezione Task - Waypoint navigation/3
  [V_vett] -> Switch di selezione Task - Waypoint navigation1/3
  [rotta_vett] -> Switch di selezione Task - Waypoint navigation3/3
  [RC_wp] -> Switch di selezione Task - Waypoint navigation/2
  [VELOCITA_wp] -> Switch di selezione Task - Waypoint navigation1/2
  [ROTTA_wp] -> Switch di selezione Task - Waypoint navigation3/2
  [V_ATO] -> Switch di selezione Task - Waypoint navigation1/4
  [RC_ATO] -> Switch di selezione Task - Waypoint navigation/4
  [rotta_ATO] -> Switch di selezione Task - Waypoint navigation3/4
  [RC_AL] -> Switch di selezione Task - Waypoint navigation/5
  [V_AL] -> Switch di selezione Task - Waypoint navigation1/5
  [rotta_AL] -> Switch di selezione Task - Waypoint navigation3/5
  [V_goHome] -> Switch di selezione Task - Waypoint navigation1/6
  [rotta_goHome] -> Switch di selezione Task - Waypoint navigation3/6
  [RC_goHome] -> Switch di selezione Task - Waypoint navigation/6
  Bus Selector/5 -> [heading]  "<heading>"
  Switch di selezione Task - Waypoint navigation2/1 -> Bus Creator2/3  "QUOTA"
  [QUOTA_wp] -> Switch di selezione Task - Waypoint navigation2/2
  [h_vett] -> Switch di selezione Task - Waypoint navigation2/3
  [h_ATO] -> Switch di selezione Task - Waypoint navigation2/4
  [h_AL] -> Switch di selezione Task - Waypoint navigation2/5
  [h_goHome] -> Switch di selezione Task - Waypoint navigation2/6
  [h] -> DECOLLO AUTOMATICO/2(h)
  [modo] -> DECOLLO AUTOMATICO/3(modo)
  [psi] -> DECOLLO AUTOMATICO/4(psi_imu)
  DECOLLO AUTOMATICO/2(Fase_ATO) -> Bus Creator/1  "Fase_ATO"
  DECOLLO AUTOMATICO/3(manetta_ref_ATO) -> Bus Creator/2  "manetta_ref_ATO"
  DECOLLO AUTOMATICO/4(eq_rot_ATO) -> Bus Creator/3  "eq_rot_ATO"
  DECOLLO AUTOMATICO/5(phi_ref_ATO) -> Bus Creator/4  "phi_ref_ATO"
  DECOLLO AUTOMATICO/6(theta_ref_ATO) -> Bus Creator/5  "theta_ref_ATO"
  Bus Creator/1 -> Inner_loop_ATO/1
  Bus Selector/8 -> [theta]  "<theta>"
  [theta] -> DECOLLO AUTOMATICO/5(theta)
  [modo] -> Chart/1(modo)
  [modo] -> Subsystem/1(modo)
  [ROTTA] -> Subsystem/2(rotta)
  [VELOCITA] -> Subsystem/3(velocita)
  [QUOTA] -> Subsystem/4(quota)
  [RC] -> Subsystem/5(RC)
  Bus Selector1/2 -> Data Type Conversion/1  "<IAS>"
  [heading] -> Subsystem/6(heading)
  Bus Selector1/3 -> Data Type Conversion1/1  "<ALT>"
  Bus Selector1/4 -> Data Type Conversion2/1  "<HDG>"
  [Tas] -> Subsystem/7(TAS)
  Bus Selector1/5 -> Data Type Conversion3/1  "<RC>"
  [h] -> Subsystem/8(h)
  Bus Selector1/6 -> Data Type Conversion4/1  "<Ingaggio_AP>"
  RC_default/1 -> Subsystem/9(RC_default)
  Subsystem/1(Out1) -> [V_vett]
  Subsystem/2(Out2) -> Scope/1, [h_vett]
  Subsystem/3(Out3) -> [rotta_vett]
  Subsystem/4(Out4) -> [RC_vett]
  Chart/4(Vec_selector) -> [Vec_selector]
  Chart/3(Go_home_selector) -> [Go_home_selector]
  Chart/2(Ato_selector) -> [Ato_selector]
  Chart/1(Al_selector) -> [Al_selector]
  Chart/5(Wp_selector) -> [Wp_selector]
  [Vec_selector] -> Subsystem/Enable
  [Lat] -> Subsystem2/1(In1)
  [Long] -> Subsystem2/2(In2)
  [h] -> Subsystem2/3(In3)
  [psi] -> Subsystem2/4(In4)
  [WP_db_info] -> Subsystem2/5(In5)
  [WP_db_param] -> Subsystem2/6(In6)
  Subsystem2/1(RC) -> [RC_wp]
  Subsystem2/2(VELOCITA) -> [VELOCITA_wp]
  Subsystem2/3(Out3) -> [QUOTA_wp]
  Subsystem2/4(Out4) -> [ROTTA_wp]
  [Wp_selector] -> Subsystem2/Enable
  [Ato_selector] -> DECOLLO AUTOMATICO/Enable
  [Lat] -> Subsystem3/1(In1)
  [Long] -> Subsystem3/2(In2)
  [h] -> Subsystem3/3(In3)
  [psi] -> Subsystem3/4(In4)
  [Lat_Home] -> Subsystem3/5(In5)
  [Long_Home] -> Subsystem3/6(In6)
  Constant/1 -> Subsystem3/7(In7)
  Constant1/1 -> Subsystem3/8(In8)
  Subsystem3/1(Out1) -> [V_goHome]
  Subsystem3/2(Out2) -> [h_goHome]
  Subsystem3/3(Out3) -> [RC_goHome]
  Subsystem3/4(Out4) -> [rotta_goHome]
  [Go_home_selector] -> Subsystem3/Enable
  Switch_attuatori/1 -> Bus Selector4/1
  Bus Selector4/1 -> AND/1  "<switch_manetta>"
  Bus Selector4/2 -> AND/2  "<switch_equilibratore>"
  Bus Selector4/4 -> AND/4  "<switch_timone>"
  Bus Selector4/3 -> AND/3  "<switch_alettoni>"
  AND/1 -> Chart/2(Ap_sel)  "Ap_sel"
  Bus Selector/9 -> [RC_sens]  "<RC>"
  [RC_sens] -> DECOLLO AUTOMATICO/6(RC)
  [Lat] -> Subsystem1/3(Lat)
  Subsystem1/5(landing_selector) -> [landing_selector]
  Subsystem1/6(H_LAT) -> [Lat_Home], H_LAT/1
  [h] -> Subsystem1/5(h)
  Subsystem1/1(TAS_AL) -> [V_AL]
  Subsystem1/3(RC_AL) -> [RC_AL]
  [Al_selector] -> Subsystem1/Enable
  Bus Selector1/1 -> Subsystem1/1(<GC_info>), Subsystem2/7(<GC_info>)  "<GC_info>"
  [Long] -> Subsystem1/4(Long)
  Subsystem1/2(QUOTA_AL) -> [h_AL]
  Subsystem1/8(H_ALT) -> H_ALT/1
  [V_] -> Subsystem1/11(V_)
  [modo] -> Subsystem1/9(modo)
  Subsystem1/4(ROTTA_AL) -> [rotta_AL]
  [Tas] -> Subsystem1/10(TAS)
  Subsystem1/7(H_LONG) -> [Long_Home], H_LONG/1
  Cal_Home/1 -> Subsystem1/2(Cal_home)
  [psi] -> Subsystem1/6(psi)
  [WP_db_info] -> Subsystem1/8(wp_db_info)
  [WP_AL] -> Subsystem1/7(wp_al)
  Bus Selector/10 -> [quota_lidar]  "<quota_lidar>"
  [quota_lidar] -> Subsystem1/12(quota_lidar)
  Data Type Conversion/1 -> Subsystem/10(<IAS>)
  Data Type Conversion1/1 -> Subsystem/11(<ALT>)
  Data Type Conversion2/1 -> Subsystem/12(<HDG>)
  Data Type Conversion3/1 -> Subsystem/13(<RC>)
  Data Type Conversion4/1 -> Subsystem/14(<Ingaggio_AP>)
  [landing_selector] -> [selector_AL], Bus Creator2/5  "landing_selector"
  Subsystem1/9(maneuver_selector) -> [maneuver_selector]
  [maneuver_selector] -> Bus Creator2/6

== system autopilota_v_15_last/scalature comandi /AILERON1 ==
  In1 : Inport
  Constant1 : Constant  Value=1503
  Gain : Gain  Gain=9
  Sum : Sum  Inputs=|++  OutDataTypeStr=double
  Out1 : Outport  VectorParamsAs1DForOutWhenUnconnected=off
  wires:
  Gain/1 -> Sum/1
  Constant1/1 -> Sum/2
  In1/1 -> Gain/1
  Sum/1 -> Out1/1

== system autopilota_v_15_last/scalature comandi /ELEVATOR1 ==
  In1 : Inport
  Constant1 : Constant  Value=3007/2
  Gain : Gain  Gain=447/50
  Sum : Sum  Inputs=|++  OutDataTypeStr=double
  Out1 : Outport  VectorParamsAs1DForOutWhenUnconnected=off
  wires:
  Gain/1 -> Sum/1
  Constant1/1 -> Sum/2
  In1/1 -> Gain/1
  Sum/1 -> Out1/1

== system autopilota_v_15_last/scalature comandi /RUDDER6 ==
  In1 : Inport
  Constant1 : Constant  Value=3007/2
  Gain : Gain  Gain=447/50
  Sum : Sum  Inputs=|++  OutDataTypeStr=double
  Out1 : Outport  VectorParamsAs1DForOutWhenUnconnected=off
  wires:
  Gain/1 -> Sum/1
  Constant1/1 -> Sum/2
  In1/1 -> Gain/1
  Sum/1 -> Out1/1

== system autopilota_v_15_last/scalature comandi /THROTTLE1 ==
  In1 : Inport
  Constant : Constant  Value=1100
  Gain : Gain  Gain=800
  Sum : Sum  Inputs=|++  OutDataTypeStr=double
  Out1 : Outport  VectorParamsAs1DForOutWhenUnconnected=off
  wires:
  In1/1 -> Gain/1
  Gain/1 -> Sum/1
  Constant/1 -> Sum/2
  Sum/1 -> Out1/1

== system autopilota_v_15_last/MISURE DA SENSORI FILTRATE/initializer//Clk_generator 1/Clock GPS1 ==
  In1 : Inport
  In2 : Inport  Port=2
  AND : Logic  Commented=on  IconShape=distinctive  AllPortsSameDT=off  OutDataTypeStr=boolean
  Equal1 : RelationalOperator  Operator===  OutDataTypeStr=boolean  RndMeth=Simplest
  From9 : From  Commented=on  GotoTag=mario
  MATLAB Function : MATLAB Function  TreatAsAtomicUnit=on
  MATLAB Function1 : MATLAB Function  TreatAsAtomicUnit=on
  Memory : Memory
  NOT : Logic  Operator=NOT  IconShape=distinctive  AllPortsSameDT=off  OutDataTypeStr=boolean
  NOT1 : Logic  Commented=on  Operator=NOT  IconShape=distinctive  AllPortsSameDT=off  OutDataTypeStr=boolean
  Pulse Generator3 : DiscretePulseGenerator  Commented=on  PulseType=Time based  Period=0.2  PulseWidth=10
  Scope : Scope
  Terminator : Terminator  Commented=on
  clk_pos : Outport  VectorParamsAs1DForOutWhenUnconnected=off
  clk_vel : Outport  Port=2  VectorParamsAs1DForOutWhenUnconnected=off
  wires:
  Equal1/1 -> NOT/1
  NOT/1 -> Scope/1, MATLAB Function1/1(u), MATLAB Function/1(u)
  In2/1 -> Equal1/1, Memory/1
  Memory/1 -> Equal1/2
  In1/1 -> MATLAB Function1/2(mario), MATLAB Function/2(mario)
  From9/1 -> NOT1/1
  Pulse Generator3/1 -> AND/1
  NOT1/1 -> AND/2
  AND/1 -> Terminator/1
  MATLAB Function1/1(y) -> clk_pos/1
  MATLAB Function/1(y) -> clk_vel/1

== system autopilota_v_15_last/MISURE DA SENSORI FILTRATE/initializer//Clk_generator 1/Clock Mti ==
  In2 : Inport
  Equal : RelationalOperator  Operator===  OutDataTypeStr=boolean  RndMeth=Simplest
  MATLAB Function : MATLAB Function  TreatAsAtomicUnit=on
  Memory : Memory
  NOT : Logic  Operator=NOT  IconShape=distinctive  AllPortsSameDT=off  OutDataTypeStr=boolean
  Out1 : Outport  VectorParamsAs1DForOutWhenUnconnected=off
  wires:
  In2/1 -> Memory/1, Equal/1
  Equal/1 -> NOT/1
  Memory/1 -> Equal/2
  MATLAB Function/1(y) -> Out1/1
  NOT/1 -> MATLAB Function/1(u)

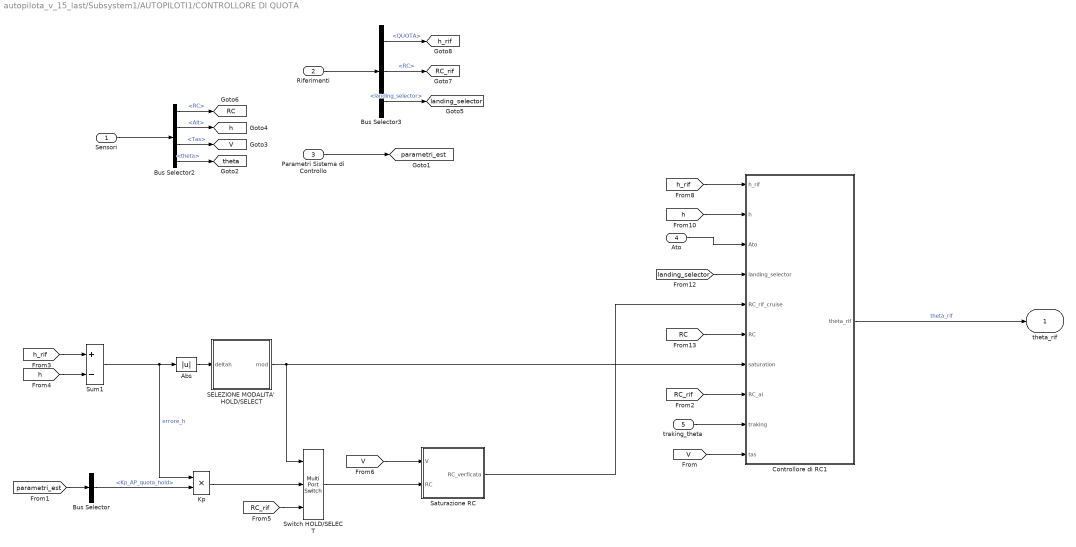
== system autopilota_v_15_last/Subsystem1/AUTOPILOTI1/CONTROLLORE DI QUOTA ==
  Sensori : Inport
  Riferimenti : Inport  Port=2
  Parametri Sistema di Controllo : Inport  Port=3
  Ato : Inport  Port=4
  traking_theta : Inport  Port=5
  Abs : Abs
  Bus Selector : BusSelector  OutputSignals=Kp_AP_quota_hold
  Bus Selector2 : BusSelector  OutputSignals=RC,Alt,Tas,theta
  Bus Selector3 : BusSelector  OutputSignals=QUOTA,RC,landing_selector
  Controllore di RC1 : Subsystem
  Kp : Product  RndMeth=Zero
  SELEZIONE MODALITA' HOLD/SELECT : Stateflow chart  TreatAsAtomicUnit=on
  "Saturazione RC " : Subsystem
  Sum1 : Sum  Inputs=+-
  Switch HOLD/SELECT : MultiPortSwitch  DataPortOrder=Zero-based contiguous  Inputs=2  zeroidx=on
  theta_rif : Outport  VectorParamsAs1DForOutWhenUnconnected=off
  tag scope: RC=global, RC_rif=global, V=global, h=global, h_rif=global, landing_selector=global, parametri_est=global, theta=global
  wires:
  Sensori/1 -> Bus Selector2/1
  Riferimenti/1 -> Bus Selector3/1
  Parametri Sistema di Controllo/1 -> [parametri_est]
  Bus Selector2/1 -> [RC]  "<RC>"
  Bus Selector2/2 -> [h]  "<Alt>"
  Bus Selector2/3 -> [V]  "<Tas>"
  Bus Selector2/4 -> [theta]  "<theta>"
  Bus Selector3/1 -> [h_rif]  "<QUOTA>"
  Bus Selector3/2 -> [RC_rif]  "<RC>"
  [V] -> "Saturazione RC "/1(V)
  Sum1/1 -> Abs/1, Kp/1  "errore_h"
  [h_rif] -> Sum1/1
  [h] -> Sum1/2
  Abs/1 -> SELEZIONE MODALITA' HOLD/SELECT/1(deltah)
  Kp/1 -> Switch HOLD/SELECT/2
  [RC_rif] -> Switch HOLD/SELECT/3
  SELEZIONE MODALITA' HOLD/SELECT/1(mod) -> Switch HOLD/SELECT/1, Controllore di RC1/7(saturation)
  [parametri_est] -> Bus Selector/1
  Bus Selector/1 -> Kp/2  "<Kp_AP_quota_hold>"
  Switch HOLD/SELECT/1 -> "Saturazione RC "/2(RC)
  Bus Selector3/3 -> [landing_selector]  "<landing_selector>"
  [h] -> Controllore di RC1/2(h)
  [h_rif] -> Controllore di RC1/1(h_rif)
  [landing_selector] -> Controllore di RC1/4(landing_selector)
  Ato/1 -> Controllore di RC1/3("Ato ")
  Controllore di RC1/1(theta_rif) -> theta_rif/1  "theta_rif"
  [RC] -> Controllore di RC1/6(RC)
  "Saturazione RC "/1(RC_verficata) -> Controllore di RC1/5(RC_rif_cruise)
  [RC_rif] -> Controllore di RC1/8("RC_al ")
  traking_theta/1 -> Controllore di RC1/9(traking)
  [V] -> Controllore di RC1/10(tas)

== system autopilota_v_15_last/Subsystem1/AUTOPILOTI1/CONTROLLORE DI ROTTA ==
  Riferimenti : Inport
  Sensori : Inport  Port=2
  Parametri Sistema di Controllo : Inport  Port=3
  "switch alettoni " : Inport  Port=4
  track_phi : Inport  Port=5
  Switch_ATO : Inport  Port=6
  ATO : Subsystem
  Bus Selector1 : BusSelector  OutputSignals=ROTTA
  Bus Selector3 : BusSelector  OutputSignals=Kp_AP_rotta,Ki_AP_rotta
  Bus Selector4 : BusSelector  OutputSignals=heading,Tas,phi,Alt,psi,v
  Constant : Constant  Value=70
  Constant2 : Constant  Value=Ki_AP_rotta
  PID Controller1 : pid_lib/PID Controller  Controller=PID  Form=Parallel  TimeDomain=Discrete-time  UseExternalTs=off  SampleTime=-1  IntegratorMethod=Forward Euler  FilterMethod=Forward Euler  ControllerParametersSource=external  P=1  I=1  D=0  UseFilter=on  N=100  TunerSelectOption=Transfer Function Based (PID Tuner App)  InitialConditionSource=internal  InitialConditionForIntegrator=0  InitialConditionForFilter=0  DifferentiatorICPrevScaledInput=0  ExternalReset=none  TrackingMode=on  Kt=1  LimitOutput=on  SatLimitsSource=internal  UpperSaturationLimit=0.7854  LowerSaturationLimit=-0.7854  LinearizeAsGain=on  AntiWindupMode=clamping  Kb=0.1  POutMin=[]  POutMax=[]  IOutMin=[]  IOutMax=[]  DOutMin=[]  DOutMax=[]  NOutMin=[]  NOutMax=[]  SumOutMin=[]  SumOutMax=[]  SaturationOutMin=[]  SaturationOutMax=[]  PParamMin=[]  PParamMax=[]  IParamMin=[]  IParamMax=[]  DParamMin=[]  DParamMax=[]  NParamMin=[]  NParamMax=[]  KbParamMin=[]  KbParamMax=[]  KtParamMin=[]  KtParamMax=[]  KbOutMin=[]  KbOutMax=[]  KtOutMin=[]  KtOutMax=[]  IntegratorOutMin=[]  IntegratorOutMax=[]  FilterOutMin=[]  FilterOutMax=[]  SumI1OutMin=[]  SumI1OutMax=[]  SumI2OutMin=[]  SumI2OutMax=[]  SumI3OutMin=[]  SumI3OutMax=[]  SumI4OutMin=[]  SumI4OutMax=[]  SumDOutMin=[]  SumDOutMax=[]  DifferentiatorOutMin=[]  DifferentiatorOutMax=[]  FilterDiffOutCoefMin=[]  FilterDiffOutCoefMax=[]  ReciprocalOutMin=[]  ReciprocalOutMax=[]  SumDenOutMin=[]  SumDenOutMax=[]  SumNumOutMin=[]  SumNumOutMax=[]  DivideOutMin=[]  DivideOutMax=[]  UdiffTsProdOutMin=[]  UdiffTsProdOutMax=[]  NTsProdOutMin=[]  NTsProdOutMax=[]  UintegralTsProdOutMin=[]  UintegralTsProdOutMax=[]  UngainTsProdOutMin=[]  UngainTsProdOutMax=[]  IntegratorContinuousStateAttributes=''  IntegratorStateMustResolveToSignalObject=off  IntegratorRTWStateStorageClass=Auto  FilterContinuousStateAttributes=''  FilterStateMustResolveToSignalObject=off  FilterRTWStateStorageClass=Auto  ParallelPVariant=ExternalParameters  IdealPVariant=Disabled  IVariant=ExternalParameters  DVariant=ExternalParameters  IntegratorVariant=Discrete  SatVariant=Enabled  AWVariant=DiscClampingParallel  PCopyVariant=Disabled  TRVariant=Enabled  FdbkBlocksVariant=Forward  IdealPFdbkVariant=Disabled  SatFdbkVariant=Disabled  DerivativeFilterVariant=ForwardEulerFilter  NVariant=ExternalParameters  NCopyVariant=Disabled  FilterICVariant=InternalICsFilter  IntegratorICVariant=InternalICs  ExternalResetVariant=Disabled  TRSumVariant=TrackingMode  SumFdbkVariant=Disabled  SumVariant=Sum_PID  TsampFilterVariant=InternalTs  TsampNgainVariant=Passthrough  TsampIntegralVariant=Passthrough  ExternalSaturationOutDataTypeStr=Inherit: Same as second input
  Switch : Switch  Criteria=u2 > Threshold  Threshold=5
  Switch auto-manual : MultiPortSwitch  DataPortOrder=Zero-based contiguous  Inputs=2  zeroidx=on
  Terminator : Terminator
  "calcolo errore Psi " : Subsystem
  phi_rif : Outport  VectorParamsAs1DForOutWhenUnconnected=off
  wires:
  Bus Selector1/1 -> "calcolo errore Psi "/1(psi_ref (°))  "<ROTTA>"
  Sensori/1 -> Bus Selector4/1
  Riferimenti/1 -> Bus Selector1/1
  Bus Selector4/1 -> [heading]  "<heading>"
  Bus Selector4/2 -> Terminator/1  "<Tas>"
  [rotta] -> "calcolo errore Psi "/2(psi (rad))
  Bus Selector4/3 -> [phi]  "<phi>"
  Parametri Sistema di Controllo/1 -> Bus Selector3/1
  "calcolo errore Psi "/1(psi_err) -> PID Controller1/1
  Constant/1 -> PID Controller1/5
  PID Controller1/1 -> Switch auto-manual/3
  Bus Selector4/4 -> [Alt]  "<Alt>"
  Bus Selector3/2 -> ATO/4(In4)  "<Ki_AP_rotta>"
  Bus Selector3/1 -> ATO/1(In1)  "<Kp_AP_rotta>"
  Constant2/1 -> PID Controller1/3
  "switch alettoni "/1 -> Switch auto-manual/1
  Bus Selector4/5 -> [psi]  "<psi>"
  Bus Selector4/6 -> [V_]  "<v>"
  [V_] -> Switch/2
  [heading] -> Switch/1
  [psi] -> Switch/3
  Switch/1 -> [rotta]
  [phi] -> Switch auto-manual/2
  Switch auto-manual/1 -> phi_rif/1
  track_phi/1 -> PID Controller1/6
  [Switch_ATO] -> ATO/2(In2)
  [Alt] -> ATO/3(In3)
  ATO/1(Out1) -> PID Controller1/2
  ATO/2("Out2 ") -> PID Controller1/4
  Switch_ATO/1 -> [Switch_ATO]

== system autopilota_v_15_last/Subsystem1/AUTOPILOTI1/CONTROLLORE DI VELOCITA' ==
  note: CANALE DI
      |  VELOCITA'
  Sensori : Inport
  Riferimenti : Inport  Port=2
  Parametri Sistema di Controllo : Inport  Port=3
  switch_manetta : Inport  Port=4
  comandi : Inport  Port=5
  Switch_AL : Inport  Port=6
  manetta_track : Inport  Port=7
  Bus Selector : BusSelector  OutputSignals=VELOCITA,QUOTA,maneuver selector
  Bus Selector1 : BusSelector  OutputSignals=Tas,Alt,quota_lidar
  Bus Selector2 : BusSelector  OutputSignals=Kp_AP_vel,Ki_AP_vel
  Bus Selector3 : BusSelector  OutputSignals=Manual_Throttle
  PID Controller : pid_lib/PID Controller  Controller=PI  Form=Parallel  TimeDomain=Discrete-time  UseExternalTs=off  SampleTime=-1  IntegratorMethod=Forward Euler  FilterMethod=Forward Euler  ControllerParametersSource=external  P=1  I=1  D=0  UseFilter=on  N=100  TunerSelectOption=Transfer Function Based (PID Tuner App)  InitialConditionSource=internal  InitialConditionForIntegrator=0  InitialConditionForFilter=0  DifferentiatorICPrevScaledInput=0  ExternalReset=none  TrackingMode=on  Kt=1  LimitOutput=on  SatLimitsSource=internal  UpperSaturationLimit=attuatore_Tmax  LowerSaturationLimit=attuatore_Tmin  LinearizeAsGain=on  AntiWindupMode=clamping  Kb=1  POutMin=[]  POutMax=[]  IOutMin=[]  IOutMax=[]  DOutMin=[]  DOutMax=[]  NOutMin=[]  NOutMax=[]  SumOutMin=[]  SumOutMax=[]  SaturationOutMin=[]  SaturationOutMax=[]  PParamMin=[]  PParamMax=[]  IParamMin=[]  IParamMax=[]  DParamMin=[]  DParamMax=[]  NParamMin=[]  NParamMax=[]  KbParamMin=[]  KbParamMax=[]  KtParamMin=[]  KtParamMax=[]  KbOutMin=[]  KbOutMax=[]  KtOutMin=[]  KtOutMax=[]  IntegratorOutMin=[]  IntegratorOutMax=[]  FilterOutMin=[]  FilterOutMax=[]  SumI1OutMin=[]  SumI1OutMax=[]  SumI2OutMin=[]  SumI2OutMax=[]  SumI3OutMin=[]  SumI3OutMax=[]  SumI4OutMin=[]  SumI4OutMax=[]  SumDOutMin=[]  SumDOutMax=[]  DifferentiatorOutMin=[]  DifferentiatorOutMax=[]  FilterDiffOutCoefMin=[]  FilterDiffOutCoefMax=[]  ReciprocalOutMin=[]  ReciprocalOutMax=[]  SumDenOutMin=[]  SumDenOutMax=[]  SumNumOutMin=[]  SumNumOutMax=[]  DivideOutMin=[]  DivideOutMax=[]  UdiffTsProdOutMin=[]  UdiffTsProdOutMax=[]  NTsProdOutMin=[]  NTsProdOutMax=[]  UintegralTsProdOutMin=[]  UintegralTsProdOutMax=[]  UngainTsProdOutMin=[]  UngainTsProdOutMax=[]  IntegratorContinuousStateAttributes=''  IntegratorStateMustResolveToSignalObject=off  IntegratorRTWStateStorageClass=Auto  FilterContinuousStateAttributes=''  FilterStateMustResolveToSignalObject=off  FilterRTWStateStorageClass=Auto  ParallelPVariant=ExternalParameters  IdealPVariant=Disabled  IVariant=ExternalParameters  DVariant=Disabled  IntegratorVariant=Discrete  SatVariant=Enabled  AWVariant=DiscClampingParallel  PCopyVariant=Disabled  TRVariant=Enabled  FdbkBlocksVariant=Forward  IdealPFdbkVariant=Disabled  SatFdbkVariant=Disabled  DerivativeFilterVariant=Disabled  NVariant=Disabled  NCopyVariant=Disabled_SignalSpec  FilterICVariant=Disabled  IntegratorICVariant=InternalICs  ExternalResetVariant=Disabled  TRSumVariant=TrackingMode  SumFdbkVariant=Disabled  SumVariant=Sum_PI  TsampFilterVariant=InternalTs  TsampNgainVariant=Passthrough  TsampIntegralVariant=Passthrough  ExternalSaturationOutDataTypeStr=Inherit: Same as second input
  Scope : Scope
  Sum3 : Sum  Inputs=-+
  Switch Bumpless 1 : MultiPortSwitch  DataPortOrder=Zero-based contiguous  Inputs=2  zeroidx=on
  Terminator : Terminator
  Terminator1 : Terminator
  Terminator2 : Terminator
  throttle - landing : Subsystem
  Riferimento Manetta : Outport  VectorParamsAs1DForOutWhenUnconnected=off
  wires:
  Sensori/1 -> Bus Selector1/1
  Riferimenti/1 -> Bus Selector/1
  Bus Selector/1 -> Sum3/2  "<VELOCITA>"
  Bus Selector1/1 -> Terminator2/1, Sum3/1  "<Tas>"
  comandi/1 -> Bus Selector3/1
  switch_manetta/1 -> [switch_manetta]
  Bus Selector1/2 -> Terminator1/1  "<Alt>"
  Parametri Sistema di Controllo/1 -> Bus Selector2/1
  Bus Selector2/1 -> PID Controller/2  "<Kp_AP_vel>"
  Bus Selector2/2 -> PID Controller/3  "<Ki_AP_vel>"
  Sum3/1 -> PID Controller/1
  PID Controller/1 -> Switch Bumpless 1/3
  Bus Selector3/1 -> [Manual_Throttle]  "<Manual_Throttle>"
  [Manual_Throttle] -> Switch Bumpless 1/2
  [switch_manetta] -> Switch Bumpless 1/1
  Switch Bumpless 1/1 -> throttle - landing/2(In2)
  [quota_al_ref] -> throttle - landing/3(Alt)
  Switch_AL/1 -> throttle - landing/1(AL)
  throttle - landing/1(Out1) -> Scope/1, Riferimento Manetta/1
  Bus Selector1/3 -> Terminator/1  "<quota_lidar>"
  Bus Selector/2 -> [quota_al_ref]  "<QUOTA>"
  manetta_track/1 -> PID Controller/4
  Bus Selector/3 -> throttle - landing/4(In4)  "<maneuver selector>"
